simulink model "model6_observer_rwp"  (R2017a)
settings: Solver=ode1  StartTime=0.0  StopTime=1000  FixedStep=0.005  RelTol=1e-3  EnableMultiTasking=on
undefined symbols (not defined in the file): A, B, C, K, L
libraries: c6xlib x2
Description:
  | Real-Time Van der Pol Simulation
  | 
  | This demonstration shows a real-time version of the Simulink(R) Van der Pol
  | simulation demo. This model does not need any external signals, so it does
  | not need any data acquisition hardware or driver. This makes the model ideal
  | for first experiments with Real-Time Windows Target(TM), without need to
  | worry about proper I/O hardware configuration.
  | 
  | How to run this demo:
  | 
  |   1. Build the model using Tools -> Real-Time Workshop -> Build Model.
  |   2. Connect to the real-time code using Simulation -> Connect to target.
  |   3. Start the real-time execution using Simulation -> Start real-time code.
settings Model: SimulationMode=external  ExtModeTrigDuration=50000  Creator=Houska  LastModifiedBy=vjdixit2
settings DataIOCC: LimitDataPoints=on  SaveFormat=Array  SignalLoggingSaveFormat=ModelDataLogs  SignalLoggingName=logsOut
settings OptimizationCC: ExpressionDepthLimit=2147483647  InitFltsAndDblsToZero=on  EfficientMapNaN2IntZero=off
settings DebuggingCC: UnderspecifiedInitializationDetection=Classic  MergeDetectMultiDrivingBlocksExec=none  SignalResolutionControl=TryResolveAllWithWarning  FcnCallInpInsideContextMsg=warning  StateNameClashWarn=warning  SFUnexpectedBacktrackingDiag=warning  SFNoUnconditionalDefaultTransitionDiag=warning  SFExecutionAtInitializationDiag=none
settings ModelReferenceCC: PropagateSignalLabelsOutOfModel=off
settings RTWCC: SystemTargetFile=sldrt.tlc  TemplateMakefile=sldrt.tmf  Description=Simulink Desktop Real-Time  RTWCompilerOptimization=on
settings CodeAppCC: MaxIdLength=95
settings SimulinkDesktopRealTimeCC: TargetPreCompLibLocation=C:\MATLABR2017a\toolbox\sldrt\lib\win64  TargetLangStandard=C89/C90 (ANSI)  SupportVariableSizeSignals=off
settings ConfigComp: CovMetricSettings=dw  CovHtmlReporting=on  CovSaveCumulativeToWorkspaceVar=on  CovSaveSingleToWorkspaceVar=on  CovExternalEMLEnable=off  CovSFcnEnable=off

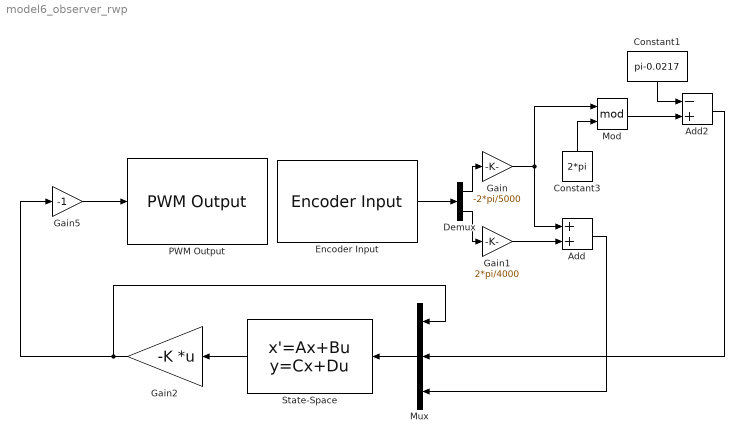
== system model6_observer_rwp ==
  Add : Sum
  Add2 : Sum  Inputs=-+
  Constant1 : Constant  Value=pi-0.0217
  Constant3 : Constant  Value=2*pi
  Demux : Demux  Outputs=2
  Encoder Input : c6xlib/Encoder Input  baseAddr=0x378  channels=[0 1]  sampleTime=str2num(get_param(bdroot, 'FixedStep'))
  Gain : Gain  Gain=-2*pi/5000
  Gain1 : Gain  Gain=2*pi/4000
  Gain2 : Gain  Gain=-K  Multiplication=Matrix(K*u)
  Gain5 : Gain  Gain=-1
  Mod : Math  Operator=mod  SaturateOnIntegerOverflow=on
  Mux : Mux  Inputs=3
  PWM Output : c6xlib/PWM Output  baseAddr=0x378  channels=0  initialOutputs=0  finalOutputs=0  sampleTime=str2num(get_param(bdroot, 'FixedStep'))
  State-Space : StateSpace  A=A-(L*C)  B=[B L]  C=eye(4)  D=zeros(4,3)  X0=0
  wires:
  Demux/2 -> Gain1/1
  Add/1 -> Mux/3
  Gain5/1 -> PWM Output/1
  Gain/1 -> Mod/1, Add/1
  Demux/1 -> Gain/1
  State-Space/1 -> Gain2/1
  Add2/1 -> Mux/2
  Encoder Input/1 -> Demux/1
  Gain1/1 -> Add/2
  Mux/1 -> State-Space/1
  Constant1/1 -> Add2/1
  Constant3/1 -> Mod/2
  Mod/1 -> Add2/2
  Gain2/1 -> Gain5/1, Mux/1
